simulink model "KayakPlant"  (R2016b)
settings: Solver=VariableStepAuto  StartTime=0.0  StopTime=20  RelTol=1e-3
libraries: simulink x1
settings Model: Creator=danoponline  LastModifiedBy=rcooper

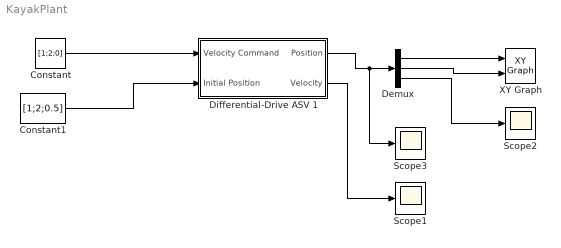
== system KayakPlant ==
  Constant : Constant  Value=[1;2;0]
  Constant1 : Constant  Value=[1;2;0.5]
  Demux : Demux  Outputs=3
  Differential-Drive ASV 1 : Subsystem
  Scope1 : Scope
  Scope2 : Scope
  Scope3 : Scope
  XY Graph : simulink/Sinks/XY Graph  xmin=0  xmax=10  ymin=0  ymax=30  st=-1
  wires:
  Constant/1 -> Differential-Drive ASV 1/1(Velocity Command)
  Constant1/1 -> Differential-Drive ASV 1/2(Initial Position)
  Differential-Drive ASV 1/1(Position) -> Scope3/1, Demux/1
  Differential-Drive ASV 1/2(Velocity) -> Scope1/1
  Demux/1 -> XY Graph/1
  Demux/2 -> XY Graph/2
  Demux/3 -> Scope2/1

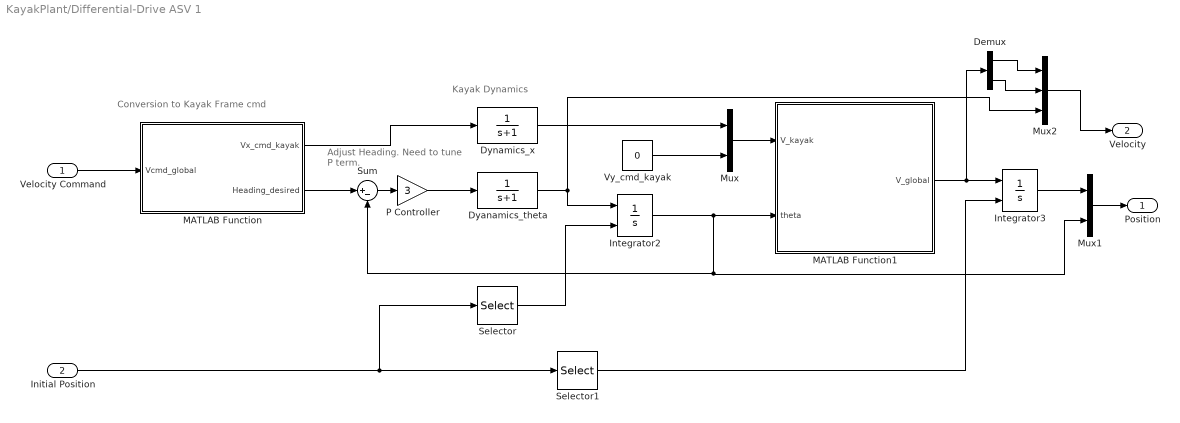
== system KayakPlant/Differential-Drive ASV 1 ==
  note: Conversion to Kayak Frame cmd
  note: Kayak Dynamics
  note: Adjust Heading. Need to tune P term.
  Velocity Command : Inport
  Initial Position : Inport  Port=2
  Demux : Demux  Outputs=2
  Dyanamics_theta : TransferFcn  Denominator=[1 1]
  Dynamics_x : TransferFcn  Denominator=[1 1]
  Integrator2 : Integrator  InitialConditionSource=external
  Integrator3 : Integrator  InitialConditionSource=external
  MATLAB Function : MATLAB Function  TreatAsAtomicUnit=on
  MATLAB Function1 : MATLAB Function  TreatAsAtomicUnit=on
  Mux : Mux  Inputs=2
  Mux1 : Mux  Inputs=2
  Mux2 : Mux  Inputs=3
  P Controller : Gain  Gain=3
  Selector : Selector  InputPortWidth=3  IndexOptions=Index vector (dialog)  Indices=[3]  OutputSizes=1
  Selector1 : Selector  InputPortWidth=3  IndexOptions=Index vector (dialog)  Indices=[1 2]  OutputSizes=1
  Sum : Sum  Inputs=|+-
  Vy_cmd_kayak : Constant  Value=0
  Position : Outport
  Velocity : Outport  Port=2
  wires:
  Velocity Command/1 -> MATLAB Function/1(Vcmd_global)
  MATLAB Function/1(Vx_cmd_kayak) -> Dynamics_x/1
  MATLAB Function/2(Heading_desired) -> Sum/1
  Sum/1 -> P Controller/1
  P Controller/1 -> Dyanamics_theta/1
  Dyanamics_theta/1 -> Mux2/3, Integrator2/1
  Initial Position/1 -> Selector1/1, Selector/1
  Mux/1 -> MATLAB Function1/1(V_kayak)
  Dynamics_x/1 -> Mux/1
  Vy_cmd_kayak/1 -> Mux/2
  Integrator2/1 -> Sum/2, Mux1/2, MATLAB Function1/2(theta)
  MATLAB Function1/1(V_global) -> Demux/1, Integrator3/1
  Selector/1 -> Integrator2/2
  Selector1/1 -> Integrator3/2
  Mux1/1 -> Position/1
  Integrator3/1 -> Mux1/1
  Demux/1 -> Mux2/1
  Demux/2 -> Mux2/2
  Mux2/1 -> Velocity/1

== matlab function KayakPlant/Differential-Drive ASV 1/MATLAB Function ==
  data: Vcmd_global input; Vx_cmd_kayak output; Heading_desired output
function [Vx_cmd_kayak,Heading_desired] = fcn(Vcmd_global)
Vx_cmd_global = Vcmd_global(1);
Vy_cmd_global = Vcmd_global(2);

Vx_cmd_kayak = sqrt(Vx_cmd_global^2 + Vy_cmd_global^2);
Heading_desired = atan2(Vy_cmd_global,Vx_cmd_global);

== matlab function KayakPlant/Differential-Drive ASV 1/MATLAB Function1 ==
  data: V_kayak input; V_global output; theta input
function V_global = Robot_to_Frame_Transformation(V_kayak,theta)
%This function calculates the local robot velocities
%based on the global robot velocities

%Initialize Variables
V_robot = [V_kayak(1);V_kayak(2)];

T = [cos(theta) -sin(theta);...
    sin(theta) cos(theta)];
V_global = T*V_robot;
